simulink model "diff_drive_extras"  (R2020b)
settings: Solver=VariableStepAuto  StartTime=0.0  StopTime=200  RelTol=1e-3
libraries: pid_lib x1, simulink x1
settings Model: Creator=Daniel  LastModifiedBy=Daniel
settings DebuggingCC: SFMachineParentedDataDiag=error

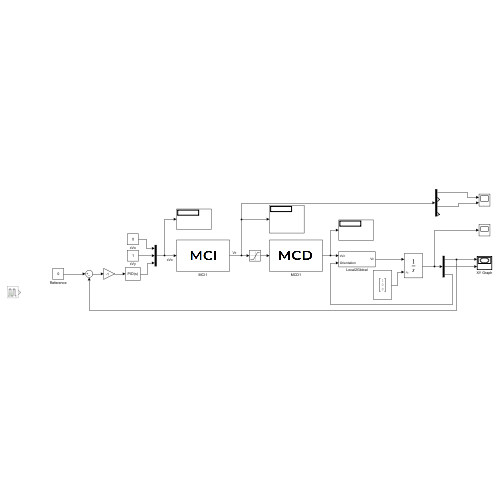
[thumbnail: Simulink's stored preview of the top-level diagram]
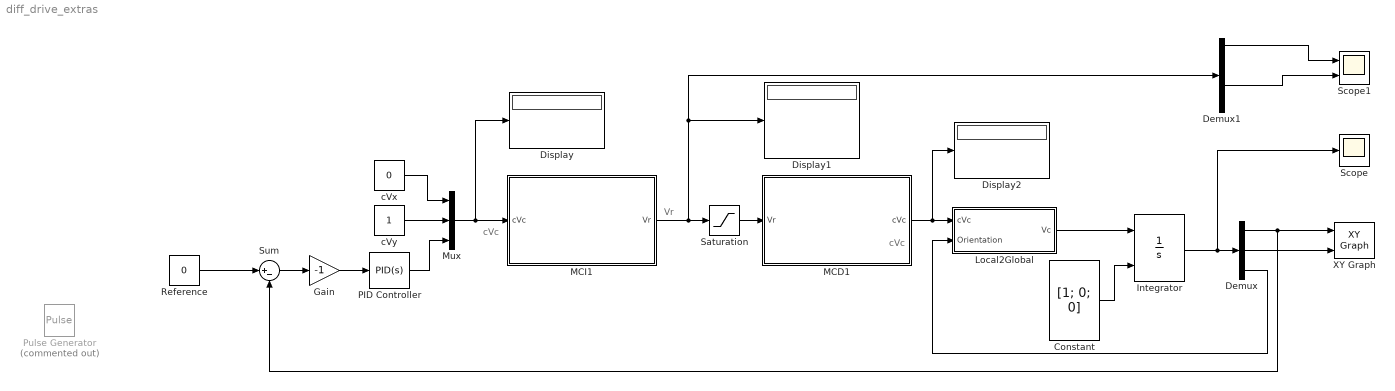
== system diff_drive_extras ==
  note: cVc
  note: Vr
  note: cVc
  Constant : Constant  Value=[1; 0; 0]  VectorParams1D=off  SampleTime=-1
  Demux : Demux  Outputs=3
  Demux1 : Demux
  Display : Display
  Display1 : Display
  Display2 : Display
  Gain : Gain  Gain=-1
  Integrator : Integrator  InitialConditionSource=external
  Local2Global : Subsystem
  MCD1 : Subsystem  mask{d1=0.05, d2=0.05}
      mask prompts: d1 "Distancia del centro a la rueda 1 (m)"; d2 "Distancia del centro a la rueda 1 (m)"
      mask Display: image('$imagefile'); % Use "Edit Image" on toolstrip to change.
  MCI1 : Subsystem  mask{d1=0.05, d2=0.05}
      mask prompts: d1 "Distancia del centro a la rueda 1 (m)"; d2 "Distancia del centro a la rueda 2 (m)"
      mask Display: image('$imagefile'); % Use "Edit Image" on toolstrip to change.
  Mux : Mux  Inputs=3
  PID Controller : pid_lib/PID Controller  Controller=PID  Form=Parallel  TimeDomain=Continuous-time  UseExternalTs=off  SampleTime=-1  IntegratorMethod=Forward Euler  FilterMethod=Forward Euler  ControllerParametersSource=internal  P=0.1  I=0.01  D=1  UseFilter=on  N=100  TunerSelectOption=Transfer Function Based (PID Tuner App)  InitialConditionSource=internal  InitialConditionForIntegrator=0  InitialConditionForFilter=0  DifferentiatorICPrevScaledInput=0  ExternalReset=none  TrackingMode=off  Kt=1  LimitOutput=off  SatLimitsSource=internal  UpperSaturationLimit=inf  LowerSaturationLimit=-inf  LinearizeAsGain=on  AntiWindupMode=none  Kb=1  POutMin=[]  POutMax=[]  IOutMin=[]  IOutMax=[]  DOutMin=[]  DOutMax=[]  NOutMin=[]  NOutMax=[]  SumOutMin=[]  SumOutMax=[]  SaturationOutMin=[]  SaturationOutMax=[]  PParamMin=[]  PParamMax=[]  IParamMin=[]  IParamMax=[]  DParamMin=[]  DParamMax=[]  NParamMin=[]  NParamMax=[]  KbParamMin=[]  KbParamMax=[]  KtParamMin=[]  KtParamMax=[]  KbOutMin=[]  KbOutMax=[]  KtOutMin=[]  KtOutMax=[]  IntegratorOutMin=[]  IntegratorOutMax=[]  FilterOutMin=[]  FilterOutMax=[]  SumI1OutMin=[]  SumI1OutMax=[]  SumI2OutMin=[]  SumI2OutMax=[]  SumI3OutMin=[]  SumI3OutMax=[]  SumI4OutMin=[]  SumI4OutMax=[]  SumDOutMin=[]  SumDOutMax=[]  DifferentiatorOutMin=[]  DifferentiatorOutMax=[]  FilterDiffOutCoefMin=[]  FilterDiffOutCoefMax=[]  ReciprocalOutMin=[]  ReciprocalOutMax=[]  SumDenOutMin=[]  SumDenOutMax=[]  SumNumOutMin=[]  SumNumOutMax=[]  DivideOutMin=[]  DivideOutMax=[]  UdiffTsProdOutMin=[]  UdiffTsProdOutMax=[]  NTsProdOutMin=[]  NTsProdOutMax=[]  UintegralTsProdOutMin=[]  UintegralTsProdOutMax=[]  UngainTsProdOutMin=[]  UngainTsProdOutMax=[]  IntegratorContinuousStateAttributes=''  IntegratorStateMustResolveToSignalObject=off  IntegratorRTWStateStorageClass=Auto  FilterContinuousStateAttributes=''  FilterStateMustResolveToSignalObject=off  FilterRTWStateStorageClass=Auto  ParallelPVariant=InternalParameters  IdealPVariant=Disabled  IVariant=InternalParameters  DVariant=InternalParameters  IntegratorVariant=Continuous  SatVariant=Disabled  AWVariant=Passthrough  PCopyVariant=Disabled  TRVariant=Disabled  FdbkBlocksVariant=Forward  IdealPFdbkVariant=Disabled  SatFdbkVariant=Disabled  DerivativeFilterVariant=ContFilter  NVariant=InternalParameters  NCopyVariant=Disabled  FilterICVariant=InternalICsFilter  IntegratorICVariant=InternalICs  ExternalResetVariant=Disabled  TRSumVariant=Passthrough  SumFdbkVariant=Disabled  SumVariant=Sum_PID  TsampFilterVariant=InternalTs  TsampNgainVariant=Passthrough  TsampIntegralVariant=Passthrough  ExternalSaturationOutDataTypeStr=Inherit: Same as second input
  Pulse Generator : DiscretePulseGenerator  Commented=on  PulseType=Time based  Period=50  PulseWidth=50
  Reference : Constant  Value=0
  Saturation : Saturate  UpperLimit=1.5  LowerLimit=-1.5
  Scope : Scope
  Scope1 : Scope  NumInputPorts=2
  Sum : Sum  Inputs=|+-
  XY Graph : simulink/Sinks/XY Graph  xmin=-1  xmax=1  ymin=-1  ymax=1  st=-1
  cVx : Constant  Value=0
  cVy : Constant
  wires:
  Mux/1 -> MCI1/1(cVc), Display/1
  cVy/1 -> Mux/2
  cVx/1 -> Mux/1
  PID Controller/1 -> Mux/3
  Constant/1 -> Integrator/2
  Integrator/1 -> Scope/1, Demux/1
  Demux/2 -> XY Graph/2
  MCI1/1(Vr) -> Demux1/1, Display1/1, Saturation/1
  MCD1/1(cVc) -> Local2Global/1(cVc), Display2/1
  Local2Global/1(Vc) -> Integrator/1
  Demux/3 -> Local2Global/2(Orientation)
  Demux1/1 -> Scope1/1
  Demux1/3 -> Scope1/2
  Sum/1 -> Gain/1
  Gain/1 -> PID Controller/1
  Demux/1 -> XY Graph/1, Sum/2
  Saturation/1 -> MCD1/1(Vr)
  Reference/1 -> Sum/1

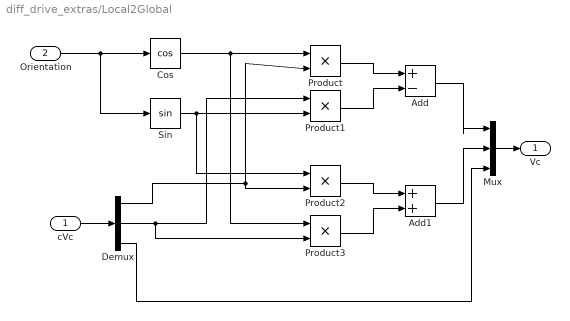
== system diff_drive_extras/Local2Global ==
  cVc : Inport
  Orientation : Inport  Port=2
  Add : Sum  Inputs=+-
  Add1 : Sum
  Cos : Trigonometry  Operator=cos
  Demux : Demux  Outputs=3
  Mux : Mux  Inputs=3
  Product{,1..3} (4 alike) : Product
  Sin : Trigonometry
  Vc : Outport
  wires:
  Orientation/1 -> Sin/1, Cos/1
  cVc/1 -> Demux/1
  Cos/1 -> Product3/1, Product/1
  Demux/1 -> Product/2, Product2/2
  Product/1 -> Add/1
  Product2/1 -> Add1/1
  Product3/1 -> Add1/2
  Demux/2 -> Product3/2, Product1/1
  Sin/1 -> Product2/1, Product1/2
  Mux/1 -> Vc/1
  Add/1 -> Mux/1
  Add1/1 -> Mux/2
  Demux/3 -> Mux/3
  Product1/1 -> Add/2

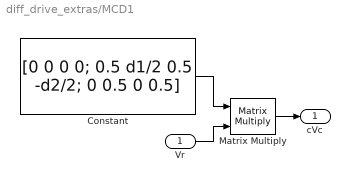
== system diff_drive_extras/MCD1 ==
  Vr : Inport
  Constant : Constant  Value=[0 0 0 0; 0.5 d1/2 0.5 -d2/2; 0 0.5 0 0.5]  VectorParams1D=off
  Matrix Multiply : Product  Multiplication=Matrix(*)
  cVc : Outport
  wires:
  Matrix Multiply/1 -> cVc/1
  Vr/1 -> Matrix Multiply/2
  Constant/1 -> Matrix Multiply/1

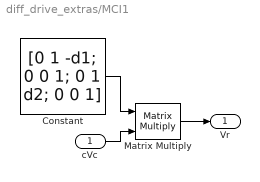
== system diff_drive_extras/MCI1 ==
  cVc : Inport
  Constant : Constant  Value=[0 1 -d1; 0 0 1; 0 1 d2; 0 0 1]  VectorParams1D=off
  Matrix Multiply : Product  Multiplication=Matrix(*)
  Vr : Outport
  wires:
  Matrix Multiply/1 -> Vr/1
  cVc/1 -> Matrix Multiply/2
  Constant/1 -> Matrix Multiply/1
